simulink model "hdlcoder_simple_counter"  (R2021a)
settings: Solver=FixedStepDiscrete  StartTime=0.0  StopTime=10.0  RelTol=1e-3
settings Model: DataTypeOverride=Off  Creator=natha  LastModifiedBy=natha
settings SolverCC: AlgebraicLoopSolver=TrustRegion
settings DataIOCC: LimitDataPoints=on  SaveOutput=off  SaveTime=off  ReturnWorkspaceOutputs=off
settings OptimizationCC: BlockReduction=off  ConditionallyExecuteInputs=off  DefaultParameterBehavior=Inlined  LifeSpan=inf
settings DebuggingCC: AlgebraicLoopMsg=error  SingleTaskRateTransMsg=error  AllowSymbolicDim=off  StrictBusMsg=ErrorOnBusTreatedAsVector  SFUnexpectedBacktrackingDiag=warning  SFNoUnconditionalDefaultTransitionDiag=warning  SFExecutionAtInitializationDiag=none  SFMachineParentedDataDiag=warning  ArithmeticOperatorsInVariantConditions=warning
settings HardwareCC: ProdBitPerPointer=32  ProdBitPerSizeT=32  ProdBitPerPtrDiffT=32  ProdLargestAtomicFloat=None  ProdIntDivRoundTo=Undefined  ProdEndianess=Unspecified  ProdWordSize=32  ProdHWDeviceType=ASIC/FPGA->ASIC/FPGA  ProdEqTarget=off
settings SFSimCC: SimUseLocalCustomCode=off  CustomCodeUndefinedFunction=UseInterfaceOnly
settings RTWCC: RTWUseLocalCustomCode=off
settings CodeAppCC: StateflowObjectComments=on
settings GRTTargetCC: TargetLangStandard=C89/C90 (ANSI)
settings ConfigComp: CovScope=ReferencedModels  CovMetricSettings=dw  CovSaveCumulativeToWorkspaceVar=on  CovSaveSingleToWorkspaceVar=on  CovExternalEMLEnable=off  CovSFcnEnable=off

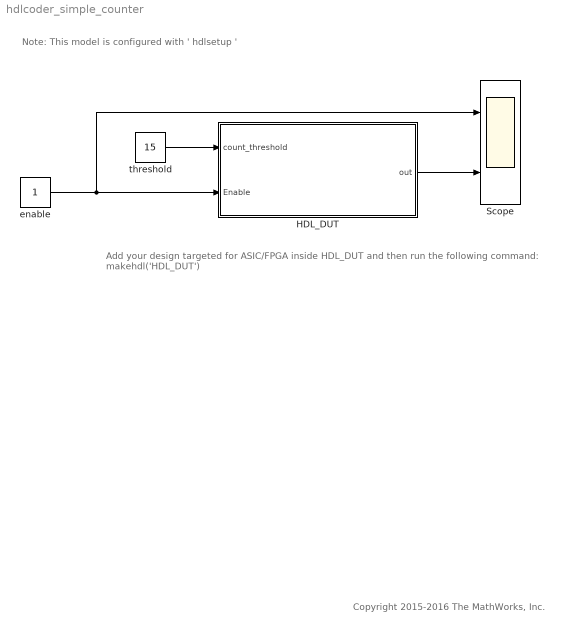
== system hdlcoder_simple_counter ==
  note: Note: This model is configured with ' hdlsetup '
  note: Add your design targeted for ASIC/FPGA inside HDL_DUT and then run the following command:
      | makehdl('HDL_DUT')
  note: Copyright 2015-2016 The MathWorks, Inc.
  HDL_DUT : Subsystem
  Scope : Scope  NumInputPorts=2
  enable : Constant  OutDataTypeStr=boolean  SampleTime=-1
  "threshold " : Constant  Value=15  OutDataTypeStr=uint8  SampleTime=-1
  wires:
  "threshold "/1 -> HDL_DUT/1("count_threshold ")
  enable/1 -> Scope/1, HDL_DUT/2(Enable)
  HDL_DUT/1(out) -> Scope/2

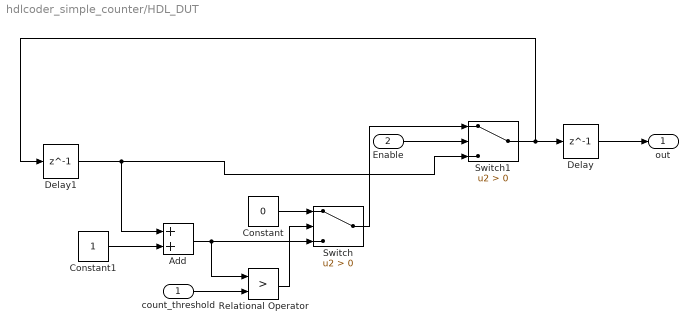
== system hdlcoder_simple_counter/HDL_DUT ==
  "count_threshold " : Inport  OutDataTypeStr=uint8
  Enable : Inport  Port=2  OutDataTypeStr=boolean
  Add : Sum  AccumDataTypeStr=uint8
  Constant : Constant  Value=0  OutDataTypeStr=uint8
  Constant1 : Constant  OutDataTypeStr=uint8
  Delay : Delay  DelayLength=1
  Delay1 : Delay  DelayLength=1
  Relational Operator : RelationalOperator  Operator=>  OutDataTypeStr=boolean  RndMeth=Nearest
  Switch : Switch  Criteria=u2 > Threshold
  Switch1 : Switch  Criteria=u2 > Threshold
  out : Outport  VectorParamsAs1DForOutWhenUnconnected=off
  wires:
  Delay/1 -> out/1
  Switch1/1 -> Delay1/1, Delay/1
  Enable/1 -> Switch1/2
  Switch/1 -> Switch1/1
  Delay1/1 -> Add/1, Switch1/3
  Add/1 -> Relational Operator/1, Switch/3
  Relational Operator/1 -> Switch/2
  "count_threshold "/1 -> Relational Operator/2
  Constant/1 -> Switch/1
  Constant1/1 -> Add/2
